simulink model "non_coherent"  (R2019b)
settings: Solver=VariableStepAuto  StartTime=0.0  StopTime=10.0  RelTol=1e-3
undefined symbols (not defined in the file): designMultirateFIR
libraries: dspmlti4 x2, dspsnks4 x1, dspvision x1, dspfdesign x1
settings Model: Creator=Siddhartha  LastModifiedBy=Siddhartha

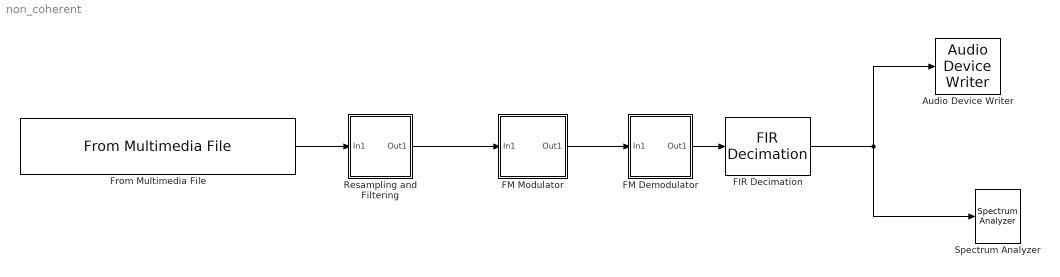
== system non_coherent ==
  Audio Device Writer : dspsnks4/Audio Device Writer  Driver=DirectSound  Device=Default  InheritSampleRate=on  SampleRate=44100  BitDepth=16-bit integer  BufferSize=4096  NumBuffers=10  DefaultOutputChannelMapping=on  OutputChannelMapping=1:2  OutputNumUnderrunSamples=off  DriverIdx=1  DeviceWarnFlag=''
  FIR Decimation : dspmlti4/FIR Decimation  FilterSource=Auto  h=designMultirateFIR(1,2)  D=5  filtStruct=Direct form  FilterObject=FDECIM  InputProcessing=Columns as channels (frame based)  framing=Enforce single-rate processing  inputOffset=0  outputBufInitCond=0  roundingMode=Floor  overflowMode=off  firstCoeffDataTypeStr=Inherit: Same word length as input  firstCoeffMin=[]  firstCoeffMax=[]  firstCoeffLastDataTypeStr=Inherit: Same word length as input  outputDataTypeStr=Inherit: Same as accumulator  outputMin=[]  outputMax=[]  outputLastDataTypeStr=Inherit: Same as accumulator
  FM Demodulator : Subsystem
  FM Modulator : Subsystem
  From Multimedia File : dspvision/From Multimedia File  inputFilename=C:\Users\Siddhartha\Desktop\Osmanthus wine tastes the same as I remember__wav(1).wav  readRange=[1 Inf]  loop=on  numPlays=inf  outputStreams=Audio only  videoDataType=single  audioDataType=double  inheritSampleTime=on  userDefinedSampleTime=1/30  noAudioOutput=off  isIntensityVideo=off  fourcc=RGB  colorVideoFormat=Separate color signals  outputEOF=off  dataOrg=Column-major  audioFrameSize=1020  computeAudioFrameSize=off  outSamplingMode=Sample based
      settings: SourceProductName=DSP System Toolbox  SourceProductBaseCode=DS
  "Resampling and Filtering " : Subsystem
  Spectrum Analyzer : SpectrumAnalyzer
  wires:
  From Multimedia File/1 -> "Resampling and Filtering "/1(In1)
  "Resampling and Filtering "/1(Out1) -> FM Modulator/1(In1)
  FM Modulator/1(Out1) -> FM Demodulator/1(In1)
  FM Demodulator/1(Out1) -> FIR Decimation/1
  FIR Decimation/1 -> Audio Device Writer/1, Spectrum Analyzer/1

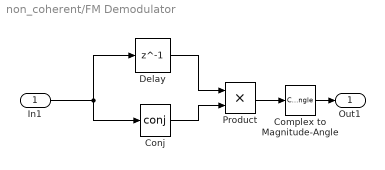
== system non_coherent/FM Demodulator ==
  In1 : Inport
  Complex to Magnitude-Angle : ComplexToMagnitudeAngle  Output=Angle
  Conj : Math  Operator=conj  SignedPower=off  SaturateOnIntegerOverflow=on
  Delay : Delay  DelayLength=1  InitialCondition=0
  Product : Product
  Out1 : Outport
  wires:
  Product/1 -> Complex to Magnitude-Angle/1
  In1/1 -> Delay/1, Conj/1
  Conj/1 -> Product/2
  Delay/1 -> Product/1
  Complex to Magnitude-Angle/1 -> Out1/1

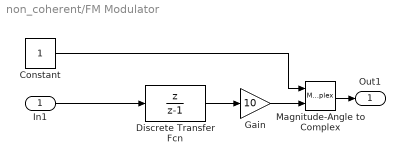
== system non_coherent/FM Modulator ==
  In1 : Inport
  Constant : Constant
  Discrete Transfer Fcn : DiscreteTransferFcn  Numerator=[1 0]  Denominator=[1 -1]
  Gain : Gain  Gain=10
  Magnitude-Angle to Complex : MagnitudeAngleToComplex
  Out1 : Outport
  wires:
  Discrete Transfer Fcn/1 -> Gain/1
  Gain/1 -> Magnitude-Angle to Complex/2
  Constant/1 -> Magnitude-Angle to Complex/1
  In1/1 -> Discrete Transfer Fcn/1
  Magnitude-Angle to Complex/1 -> Out1/1

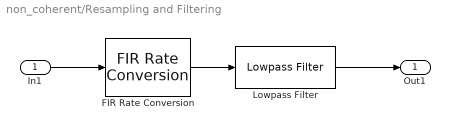
== system non_coherent/Resampling and Filtering  ==
  In1 : Inport
  FIR Rate Conversion : dspmlti4/FIR Rate Conversion  FilterSource=Auto  L=5  h=designMultirateFIR(3,2)  M=2  FilterObject=FRC  roundingMode=Floor  overflowMode=off  firstCoeffDataTypeStr=Inherit: Same word length as input  firstCoeffMin=[]  firstCoeffMax=[]  firstCoeffLastDataTypeStr=Inherit: Same word length as input  outputDataTypeStr=Inherit: Same as accumulator  outputMin=[]  outputMax=[]  outputLastDataTypeStr=Inherit: Same as accumulator
      settings: SourceProductName=DSP System Toolbox  SourceProductBaseCode=DS
  Lowpass Filter : dspfdesign/Lowpass Filter  FilterType=FIR  DesignForMinimumOrder=on  FilterOrder=50  PassbandFrequency=15e3  StopbandFrequency=20e3  PassbandRipple=0.1  StopbandAttenuation=80  InheritSampleRate=on  SampleRate=44100  SimulateUsing=Interpreted execution  roundingMode=Floor  coeffsDataTypeStr=fixdt(1,16)
  Out1 : Outport
  wires:
  FIR Rate Conversion/1 -> Lowpass Filter/1
  In1/1 -> FIR Rate Conversion/1
  Lowpass Filter/1 -> Out1/1
